simulink model "Stop"  (R2017b)
settings: Solver=FixedStepAuto  StartTime=0.0  StopTime=10.0  RelTol=1e-3  EnableMultiTasking=on
values from neighbouring files (symbols this model uses):
  K = acker(s1z.a, s1z.b, [0.2225 0.9743 0.987 0.987])    [model.m]
  K_PWM = 8.087    [model.m]
  l = 0.125    [model.m]
  R = 0.027    [model.m]
  Ts = 0.0033    [model.m]
undefined symbols (not defined in the file or in its folder): DiscIntNeverNeededParam
libraries: legoev3lib x6, simulink x1
settings Model: ExtModeTrigDuration=2  Creator=USER  LastModifiedBy=USER
settings SolverCC: PositivePriorityOrder=on
settings OptimizationCC: PassReuseOutputArgsAs=Individual arguments  MaxStackSize=64
settings DebuggingCC: ParameterTunabilityLossMsg=error
settings HardwareCC: ProdBitPerPointer=32  ProdBitPerSizeT=32  ProdBitPerPtrDiffT=32  ProdLargestAtomicInteger=Long  ProdWordSize=32  ProdHWDeviceType=ARM Compatible->ARM 9
settings SFSimCC: MATLABDynamicMemAlloc=off
settings RTWCC: SystemTargetFile=ert.tlc  HardwareBoard=LEGO MINDSTORMS EV3  TemplateMakefile=ert_default_tmf  GenerateReport=on  Toolchain=Sourcery G++ Lite v2009q3  IncludeHyperlinkInReport=on  LaunchReport=on  GenerateTraceInfo=on  GenerateTraceReport=on  GenerateTraceReportSl=on  GenerateTraceReportSf=on  GenerateTraceReportEml=on
settings CodeAppCC: ForceParamTrailComments=on  IgnoreCustomStorageClasses=off  OperatorAnnotations=on  SimulinkDataObjDesc=on  SFDataObjDesc=on  InsertBlockDesc=on
settings ERTTargetCC: SupportContinuousTime=on  SupportVariableSizeSignals=on

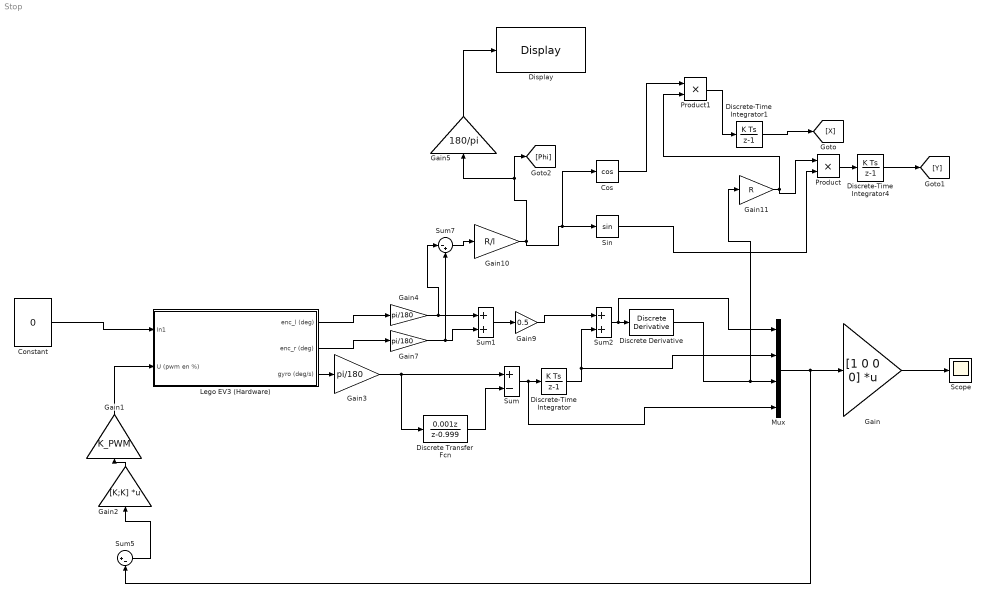
== system Stop ==
  Constant : Constant  Value=0
  Cos : Trigonometry  Operator=cos
  Discrete Transfer Fcn : DiscreteTransferFcn  Numerator=[0.001 0]  Denominator=[1 -0.999]  SampleTime=Ts
  Discrete Derivative : simulink/Discrete/Discrete Derivative  gainval=1.0  ICPrevScaledInput=0.0  OutMin=[]  OutMax=[]  OutDataType=fixdt(1, 16)  OutScaling=2^-10  DoSatur=off
  Discrete-Time Integrator : DiscreteIntegrator  InitialConditionSetting=State (most efficient)  SampleTime=Ts  ICPrevOutput=DiscIntNeverNeededParam  ICPrevScaledInput=DiscIntNeverNeededParam
  Discrete-Time Integrator1 : DiscreteIntegrator  InitialConditionSetting=State (most efficient)  SampleTime=Ts  ICPrevOutput=DiscIntNeverNeededParam  ICPrevScaledInput=DiscIntNeverNeededParam
  Discrete-Time Integrator4 : DiscreteIntegrator  InitialConditionSetting=State (most efficient)  SampleTime=Ts  ICPrevOutput=DiscIntNeverNeededParam  ICPrevScaledInput=DiscIntNeverNeededParam
  Display : legoev3lib/Display  slcdLine=1  slcdFormat=Decimal
      settings: SourceProductName=Simulink Support Package for LEGO MINDSTORMS EV3 Hardware  SourceProductBaseCode=LEGOEV3
  Gain : Gain  Gain=[1 0 0 0]  Multiplication=Matrix(K*u)
  Gain1 : Gain  Gain=K_PWM
  Gain10 : Gain  Gain=R/l
  Gain11 : Gain  Gain=R
  Gain2 : Gain  Gain=[K;K]  Multiplication=Matrix(K*u)
  Gain3 : Gain  Gain=pi/180
  Gain4 : Gain  Gain=pi/180
  Gain5 : Gain  Gain=180/pi
  Gain7 : Gain  Gain=pi/180
  Gain9 : Gain  Gain=0.5
  Lego EV3 (Hardware) : Subsystem
  Mux : Mux
  Product : Product
  Product1 : Product
  Scope : Scope
  Sin : Trigonometry
  Sum : Sum  Inputs=+-
  Sum1 : Sum
  Sum2 : Sum
  Sum5 : Sum  Inputs=|+-
  Sum7 : Sum  Inputs=|-+
  wires:
  Gain7/1 -> Sum7/2, Sum1/2
  Discrete Derivative/1 -> Gain11/1, Mux/3
  Discrete Transfer Fcn/1 -> Sum/2
  Lego EV3 (Hardware)/3(gyro (deg/s)) -> Gain3/1
  Lego EV3 (Hardware)/1(enc_l (deg)) -> Gain4/1
  Sin/1 -> Product/2
  Lego EV3 (Hardware)/2(enc_r (deg)) -> Gain7/1
  Sum5/1 -> Gain2/1
  Sum1/1 -> Gain9/1
  Gain9/1 -> Sum2/1
  Gain2/1 -> Gain1/1
  Cos/1 -> Product1/1
  Mux/1 -> Sum5/2, Gain/1
  Gain1/1 -> Lego EV3 (Hardware)/2(U (pwm en %))
  Product/1 -> Discrete-Time Integrator4/1
  Discrete-Time Integrator1/1 -> [X]
  Product1/1 -> Discrete-Time Integrator1/1
  Gain4/1 -> Sum7/1, Sum1/1
  Discrete-Time Integrator4/1 -> [Y]
  Gain11/1 -> Product/1, Product1/2
  Sum/1 -> Mux/4, Discrete-Time Integrator/1
  Discrete-Time Integrator/1 -> Mux/2, Sum2/2
  Gain/1 -> Scope/1
  Sum2/1 -> Mux/1, Discrete Derivative/1
  Sum7/1 -> Gain10/1
  Gain3/1 -> Discrete Transfer Fcn/1, Sum/1
  Gain10/1 -> Cos/1, Sin/1, Gain5/1, [Phi]
  Gain5/1 -> Display/1
  Constant/1 -> Lego EV3 (Hardware)/1(In1)

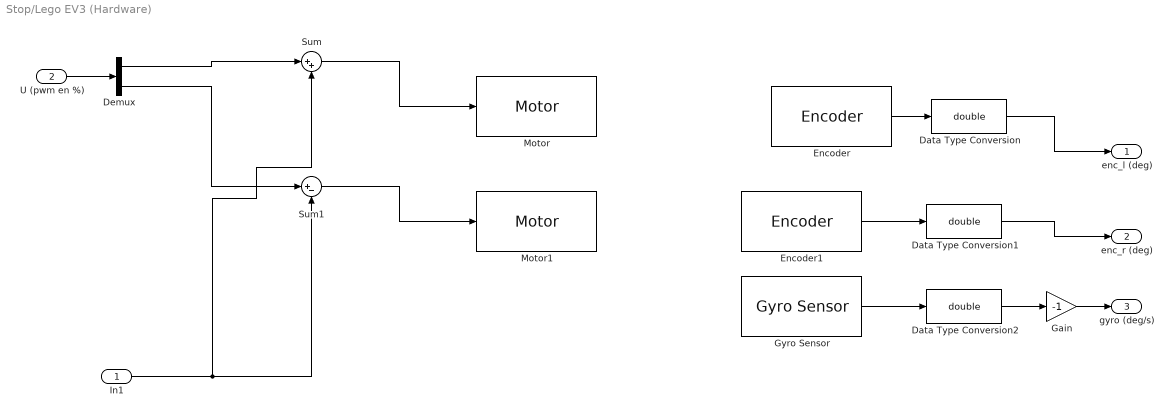
== system Stop/Lego EV3 (Hardware) ==
  In1 : Inport
  U (pwm en %) : Inport  Port=2
  Data Type Conversion : DataTypeConversion  OutDataTypeStr=double
  Data Type Conversion1 : DataTypeConversion  OutDataTypeStr=double
  Data Type Conversion2 : DataTypeConversion  OutDataTypeStr=double
  Demux : Demux  Outputs=2
  Encoder : legoev3lib/Encoder  portNumber=D  opMode=No reset  sampleTime=Ts
      settings: SourceProductName=Simulink Support Package for LEGO MINDSTORMS EV3 Hardware  SourceProductBaseCode=LEGOEV3
  Encoder1 : legoev3lib/Encoder  portNumber=A  opMode=No reset  sampleTime=Ts
      settings: SourceProductName=Simulink Support Package for LEGO MINDSTORMS EV3 Hardware  SourceProductBaseCode=LEGOEV3
  Gain : Gain  Gain=-1
  Gyro Sensor : legoev3lib/Gyro Sensor  portNumber=3  sampleTime=Ts
      settings: SourceProductName=Simulink Support Package for LEGO MINDSTORMS EV3 Hardware  SourceProductBaseCode=LEGOEV3
  Motor : legoev3lib/Motor  sportNumber=D  sstopAction=Brake
  Motor1 : legoev3lib/Motor  sportNumber=A  sstopAction=Brake
  Sum : Sum  Inputs=|++
  Sum1 : Sum  Inputs=|+-
  enc_l (deg) : Outport  VectorParamsAs1DForOutWhenUnconnected=on
  enc_r (deg) : Outport  Port=2  VectorParamsAs1DForOutWhenUnconnected=on
  gyro (deg/s) : Outport  Port=3  VectorParamsAs1DForOutWhenUnconnected=on
  wires:
  Gyro Sensor/1 -> Data Type Conversion2/1
  Encoder1/1 -> Data Type Conversion1/1
  Encoder/1 -> Data Type Conversion/1
  Data Type Conversion/1 -> enc_l (deg)/1
  Data Type Conversion1/1 -> enc_r (deg)/1
  Data Type Conversion2/1 -> Gain/1
  Gain/1 -> gyro (deg/s)/1
  U (pwm en %)/1 -> Demux/1
  Demux/1 -> Sum/1
  Demux/2 -> Sum1/1
  Sum/1 -> Motor/1
  Sum1/1 -> Motor1/1
  In1/1 -> Sum/2, Sum1/2
